simulink model "OpenSeesPy_Simulink"  (R2021a)
settings: Solver=ode8  StartTime=0.0  StopTime=31.2  FixedStep=dtfast  RelTol=1e-3
PreLoadFcn:
  | initializeSimulation;
InitFcn:
  | clear('all');
  | initializeSimulation;
undefined symbols (not defined in the file): adaptive, Area, areaC, asiv, Be, Cl, coef, damperA, damperB, damperC, damperCanon, denfilter, DiscIntNeverNeededParam, dtsim, f, fir_coef, flowCanon, forceCanon, forgfact, frictionA, frictionB, frictionC, gasConstant, Gsnsr_DT, Gsnsr_FT, Kc, ke, kgap, khard, Kp, Kq, kv, learningrate, lengthCanon, massA, massB, massC, massCanon, maxDisplA, maxDisplB, maxDisplC, maxForceC, maxOilVolume, maxVelocA, maxVelocB, maxVelocC, minDisplA, minDisplB, minDisplC, minVelocA, minVelocB, minVelocC, n1siv, n2siv, Ngap, nsiv, numfilter, P_corr_i, precharge, pumpFlow ... (+25)
libraries: simulink x4, instrumentlib x2, dsparch4 x1, sldrtlib x1
(part 1 of 3)
settings Model: Creator=diego.mera  LastModifiedBy=diego.mera
settings SolverCC: PositivePriorityOrder=on
settings OptimizationCC: EnhancedBackFolding=on  PassReuseOutputArgsAs=Individual arguments  ZeroExternalMemoryAtStartup=off  ZeroInternalMemoryAtStartup=off  MaxStackSize=64  OptimizeBlockOrder=speed  DifferentSizesBufferReuse=on  OptimizationCustomize=off  EfficientTunableParamExpr=on
settings DebuggingCC: ParameterTunabilityLossMsg=error
settings HardwareCC: ProdBitPerPointer=32  ProdBitPerSizeT=32  ProdBitPerPtrDiffT=32  ProdLargestAtomicInteger=Long  ProdLargestAtomicFloat=Double  ProdWordSize=32  ProdLongLongMode=on  ProdHWDeviceType=ARM Compatible->ARM Cortex
settings RTWCC: SystemTargetFile=ert.tlc  HardwareBoard=Raspberry Pi  TLCOptions="-aInlineSetEventsForThisBaseRateFcn=TLC_FALSE -aSuppressMultiTaskScheduler=TLC_FALSE  -aRateBasedStepFcn=0"  TemplateMakefile=ert_default_tmf  Toolchain=GNU GCC Embedded Linux  BuildConfiguration=Faster Runs
settings CodeAppCC: ForceParamTrailComments=on  IgnoreCustomStorageClasses=off  OperatorAnnotations=on  SimulinkDataObjDesc=on  SFDataObjDesc=on  InsertBlockDesc=on
settings ERTTargetCC: SupportVariableSizeSignals=on  ExtModeTransport=2  ExtModeStaticAlloc=on  ExtModeMexFile=ext_xcp  ExtModeIntrfLevel=Level2 - Open

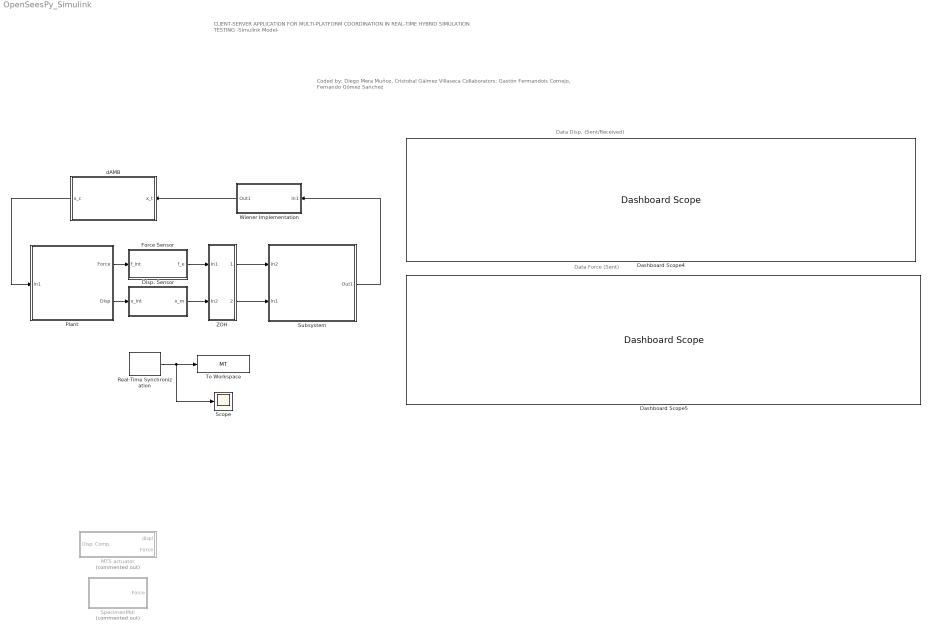
== system OpenSeesPy_Simulink ==
  note: Data Disp. (Sent/Received)
  note: Data Force (Sent)
  note: CLIENT-SERVER APPLICATION FOR MULTI-PLATFORM COORDINATION IN REAL-TIME HYBRID SIMULATION TESTING
      | -Simulink Model-
  note: Coded by: Diego Mera Muñoz, Cristobal Gálmez Villaseca
      | Collaborators: Gastón Fermandois Cornejo, Fernando Gómez Sanchez
  Dashboard Scope4 : DashboardScope  Ymin=-5  Ymax=5
  Dashboard Scope5 : DashboardScope  Ymin=-1.5e-5  Ymax=1e-5
  Disp. Sensor : Subsystem
      mask Display: disp('DISP. SENSOR')
  Force Sensor : Subsystem
      mask Display: disp('FORCE SENSOR')
  MTS actuator : Subsystem  Commented=on
  Plant : Subsystem
      mask Display: disp('PLANT\n(Actuator-ES)')
  Real-Time Synchronization : sldrtlib/Real-Time Synchronization  SampleTime=dtsim  MaxMissedTicks=1000000  ShowMissedTicks=on  YieldWhenWaiting=off
  Scope : Scope
  SpecimenMdl : Subsystem  Commented=on
      mask Display: disp('EXPERIMENTAL\nSUBSTRUCTURE')
  Subsystem : Subsystem
      mask Display: disp('NUMERICAL\nSUBSTRUCTURE')
  To Workspace : ToWorkspace  VariableName=MT  SaveFormat=Timeseries  SampleTime=-1
  Wiener Implementation : Subsystem
      mask Display: disp('MBMRT FILTER')
  ZOH : Subsystem
      mask Display: disp('ZOH')
  dAMB : Subsystem
      mask Display: disp('DISCRETE ADAPTIVE\nMODEL-BASED\nCOMPENSATION')
  wires:
  Subsystem/1(Out1) -> Wiener Implementation/1(In1)
  dAMB/1(x_c) -> Plant/1(In1)
  Real-Time Synchronization/1 -> Scope/1, To Workspace/1
  Wiener Implementation/1(Out1) -> dAMB/1(x_t)
  Plant/1(Force) -> Force Sensor/1(f_int)
  Force Sensor/1("f_e ") -> ZOH/1(In1)
  ZOH/1(Out1) -> Subsystem/1(In2)
  ZOH/2(Out2) -> Subsystem/2(In1)
  Disp. Sensor/1(x_m) -> ZOH/2(In2)
  Plant/2(Disp) -> Disp. Sensor/1(x_int)

== system OpenSeesPy_Simulink/Disp. Sensor ==
  x_int : Inport
  Sensor Noise : simulink/Sources/Band-Limited White Noise  Cov=rms_noise_DT  Ts=dtsim  seed=double(Seed_snr.Seed)
  Sensor Gain LVDT : Gain  Gain=Gsnsr_DT  SaturateOnIntegerOverflow=on  OutDataTypeStr=Inherit: Same as input  ParamDataTypeStr=Inherit: Same as input
  Sum : Sum  Inputs=|++  InputSameDT=on  SaturateOnIntegerOverflow=on  OutDataTypeStr=Inherit: Same as first input
  x_m : Outport
  tag scope: x_m=global
  wires:
  Sensor Noise/1 -> Sum/2
  Sum/1 -> x_m/1, [x_m]  "x_m"
  x_int/1 -> Sensor Gain LVDT/1
  Sensor Gain LVDT/1 -> Sum/1

== system OpenSeesPy_Simulink/Force Sensor ==
  f_int : Inport
  Sensor Noise1 : simulink/Sources/Band-Limited White Noise  Cov=rms_noise_FT  Ts=dtsim  seed=double(Seed_snr.Seed)
  Sensor Gain LOAD CELL : Gain  Gain=Gsnsr_FT  SaturateOnIntegerOverflow=on  OutDataTypeStr=Inherit: Same as input  ParamDataTypeStr=Inherit: Same as input
  Sum1 : Sum  Inputs=|++  InputSameDT=on  SaturateOnIntegerOverflow=on  OutDataTypeStr=Inherit: Same as first input
  "f_e " : Outport
  wires:
  f_int/1 -> Sensor Gain LOAD CELL/1
  Sensor Noise1/1 -> Sum1/2
  Sum1/1 -> "f_e "/1
  Sensor Gain LOAD CELL/1 -> Sum1/1

== system OpenSeesPy_Simulink/MTS actuator ==
  note: Force
  Disp. Comp. : Inport
  Analog Filter Design : dsparch4/Analog Filter Design  method=Butterworth  filttype=Lowpass  N=1  Wlo=20  Whi=80  Rp=2  Rs=40
  Proportional Gain : Gain  Gain=maxForceC/areaC
  Subtract : Sum  Inputs=+-
  accumulators : Subsystem
  dynamic long channel #1 : Subsystem
  dynamic long channel #2 : Subsystem  Commented=on
  dynamic short channel #1 : Subsystem  Commented=on
  dynamic short channel #2 : Subsystem  Commented=on
  static channel #1 : Subsystem  Commented=on
  static channel #2 : Subsystem  Commented=on
  static channel #3 : Subsystem  Commented=on
  static channel #4 : Subsystem  Commented=on
  displ : Outport
  Force : Outport  Port=2
  wires:
  Disp. Comp./1 -> Subtract/1
  Subtract/1 -> Proportional Gain/1
  dynamic long channel #1/3(flow) -> accumulators/1(flow)
  dynamic long channel #1/2(force) -> Analog Filter Design/1
  dynamic long channel #1/1(displ) -> displ/1, Subtract/2
  accumulators/1(press) -> dynamic long channel #1/2(spl press)
  Analog Filter Design/1 -> Force/1
  Proportional Gain/1 -> dynamic long channel #1/1(valve cmd)

== system OpenSeesPy_Simulink/Plant ==
  note: Modeling of Actuator Dynamics
  In1 : Inport
  Actuator : TransferFcn  Denominator=[Vt/(4*Be) Cl]
      mask Display: image(imread('actuator.PNG'));
  Controller : Gain  Gain=Kp
  Gain1 : Gain  Gain=Area
  Gain2 : Gain  Gain=Area
  Scope1 : Scope
  Servovalve Dynamics : TransferFcn  Numerator=[kv]  Denominator=[tauv 1]
      mask Display: image(imread('servo2.PNG'));
  Servovalve Flow : Subsystem
      settings: PortSchema="{\"entries\":[{\"content\":{\"sides\":[{\"content\":{\"connectorIds\":[\"In1\"]},\"type\":\"ConnectorPlacement.EquallySpacedRectSide\",\"uuid\":\"f3a8b7d5-d784-462c-bc82-60644eee5a75\"},{\"content\":{\"connectorIds\":[\"Out1\"],\"side\":\"RIGHT\"},\"type\":\"ConnectorPlacement.EquallySpacedRectSide\",\"uuid\":\"5e6f1f83-a632-4bc9-a761-43cae998e77f\"},{\"content\":{\"connectorIds\":[\"In2\"],\"side\":\"TOP\"},\"type\":\"ConnectorPlacement.EquallySpacedRectSide\",\"uuid\":\"989b0903-e260-4847-946f-0ac5d5e511f7\"}]},\"type\":\"ConnectorPlacement.EquallySpacedConnector\",\"uuid\":\"5619e211-faa3-4076-b1a0-b20862ba0eaa\"}],\"packageUris\":[\"http://schema.mathworks.com/mf0/Connector/19700101\"],\"version\":\"1.0\"}"
      mask Display: image(imread('servo.PNG'));
  Subsystem : Subsystem
      mask Display: disp('EXPERIMENTAL\nSUBSTRUCTURE')
  Sum : Sum  Inputs=|+-
  Sum1 : Sum  Inputs=|+-
  To Workspace : ToWorkspace  VariableName=Force_act  SaveFormat=Timeseries  SampleTime=-1
  Force : Outport
  Disp : Outport  Port=2
  wires:
  Sum/1 -> Controller/1  "e"
  Servovalve Dynamics/1 -> Servovalve Flow/1(xv)  "x_v"
  Gain1/1 -> Sum1/2  "caudal"
  Actuator/1 -> Servovalve Flow/2(pL), Gain2/1  "PL"
  Sum1/1 -> Actuator/1
  Controller/1 -> Servovalve Dynamics/1  "i_c"
  Servovalve Flow/1(QL) -> Sum1/1
  Gain2/1 -> Subsystem/1(F), To Workspace/1, Scope1/1, Force/1  "f_p"
  Subsystem/2(x_m s) -> Gain1/1
  Subsystem/1(x_m) -> Disp/1, Sum/2
  In1/1 -> Sum/1

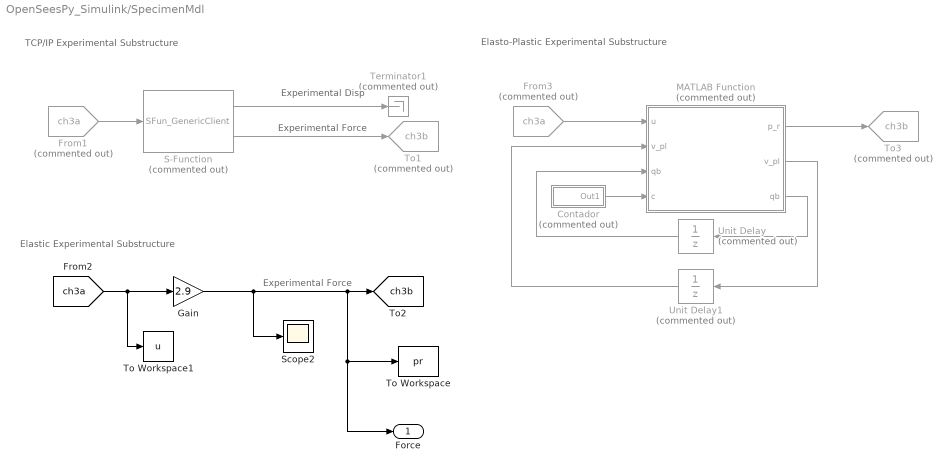
== system OpenSeesPy_Simulink/SpecimenMdl ==
  note: Elasto-Plastic Experimental Substructure
  note: Elastic Experimental Substructure
  note: Experimental Force
  note: Experimental Disp
  note: TCP/IP Experimental Substructure
  note: Experimental Force
  Contador : Subsystem  Commented=on
      mask Display: disp('Contador')
  From1 : From  Commented=on  GotoTag=ch3a  TagVisibility=global
  From3 : From  Commented=on  GotoTag=ch3a  TagVisibility=global
  Gain : Gain  Gain=2.9
  MATLAB Function : MATLAB Function  Commented=on  TreatAsAtomicUnit=on
  S-Function : S-Function  Commented=on  FunctionName=SFun_GenericClient  Parameters=ipAddr,ipPort,dataSize  SFunctionDeploymentMode=off  EnableBusSupport=off  mask(GenericClient Element){ipAddr=127.0.0.1, ipPort=8093, dataSize=256}
      mask prompts: ipAddr "IP Address of Server"; ipPort "IP Port Number of Server"; dataSize "Size of Data Arrays"
      mask Display: disp('GenericClient\nElement');
  Scope2 : Scope
  Terminator1 : Terminator  Commented=on
  To Workspace : ToWorkspace  VariableName=pr  SaveFormat=Timeseries  SampleTime=-1
  To Workspace1 : ToWorkspace  VariableName=u  SaveFormat=Timeseries  SampleTime=-1
  To1 : Goto  Commented=on  GotoTag=ch3b  TagVisibility=global
  To3 : Goto  Commented=on  GotoTag=ch3b  TagVisibility=global
  Unit Delay : UnitDelay  Commented=on  SampleTime=-1  HasFrameUpgradeWarning=on
  Unit Delay1 : UnitDelay  Commented=on  SampleTime=-1  HasFrameUpgradeWarning=on
  Force : Outport
  tag scope: ch3b=global
  wires:
  [ch3a] -> To Workspace1/1, Gain/1
  Gain/1 -> To Workspace/1, Force/1, [ch3b], Scope2/1
  From3/1 -> MATLAB Function/1(u)
  MATLAB Function/3(qb) -> Unit Delay/1
  MATLAB Function/1(p_r) -> To3/1
  Unit Delay/1 -> MATLAB Function/3("qb ")
  Contador/1(Out1) -> MATLAB Function/4(c)
  MATLAB Function/2(v_pl) -> Unit Delay1/1
  Unit Delay1/1 -> MATLAB Function/2("v_pl ")
  From1/1 -> S-Function/1
  S-Function/2 -> To1/1
  S-Function/1 -> Terminator1/1

== system OpenSeesPy_Simulink/Subsystem ==
  In2 : Inport
  In1 : Inport  Port=2
  TCP/IP Receive5 : instrumentlib/TCP//IP Receive  Priority=1  Host=127.0.0.1  Port=8090  DataSize=1  EnableBlockingMode=off  Timeout=10  SampleTime=dtsim  DataType=double  ByteOrder=BigEndian  ASCIIFormatting=%f,  Terminator=LF
  TCP/IP Send5 : instrumentlib/TCP//IP Send  Priority=2  Host=127.0.0.1  Port=8090  EnableBlockingMode=off  Timeout=0.02  ByteOrder=BigEndian  TransferDelay=on
  Terminator : Terminator
  To Workspace : ToWorkspace  VariableName=Disp_Num  SaveFormat=Timeseries  SampleTime=-1
  Out1 : Outport
  wires:
  In1/1 -> Terminator/1
  In2/1 -> TCP/IP Send5/1
  TCP/IP Receive5/1 -> To Workspace/1, Out1/1

== system OpenSeesPy_Simulink/Wiener Implementation ==
  In1 : Inport
  Prediction_Adaptive_Fixed : Subsystem
      mask Display: disp('PREDICTION\n(Adaptive/Fixed w)')
  Test3 : Subsystem
      mask Display: disp('MONOMIAL\nINTERPOLATION')
  To Workspace : ToWorkspace  VariableName=adaptive_parameters  SaveFormat=Timeseries  SampleTime=-1
  Out1 : Outport
  wires:
  Test3/1(Out1) -> Out1/1
  In1/1 -> Prediction_Adaptive_Fixed/1(In1)
  Prediction_Adaptive_Fixed/2(Out2) -> To Workspace/1
  Prediction_Adaptive_Fixed/1(Out1) -> Test3/1(In1)

== system OpenSeesPy_Simulink/ZOH ==
  In1 : Inport
  In2 : Inport  Port=2
  Rate Transition : RateTransition  OutPortSampleTime=dtsim
  Rate Transition1 : RateTransition  OutPortSampleTime=dtsim
  Out1 : Outport
  Out2 : Outport  Port=2
  wires:
  In1/1 -> Rate Transition/1  "Force_Num"
  In2/1 -> Rate Transition1/1  "Disp_Num"
  Rate Transition/1 -> Out1/1
  Rate Transition1/1 -> Out2/1

== system OpenSeesPy_Simulink/dAMB ==
  x_t : Inport
  Discrete Transfer Fcn : DiscreteTransferFcn  Numerator=[numfilter]  Denominator=[denfilter]
  Discrete Transfer Fcn1 : DiscreteTransferFcn  Numerator=[numfilter]  Denominator=[denfilter]
  Dot Product : DotProduct  InputSameDT=on  OutDataTypeStr=Inherit: Inherit via internal rule
  Gain : Gain  Gain=0.0254
  Gain1 : Gain  Gain=0.0254
  Gain2 : Gain  Gain=39.3701
  RLS : Subsystem
  Tapped Delay : simulink/Discrete/Tapped Delay  vinit=0.0  samptime=-1  NumDelays=fir_coef-1  DelayOrder=Newest  includeCurrent=on
  Tapped Delay1 : simulink/Discrete/Tapped Delay  vinit=0.0  samptime=-1  NumDelays=fir_coef-1  DelayOrder=Newest  includeCurrent=on
  To Workspace : ToWorkspace  VariableName=x_t  SaveFormat=Timeseries  SampleTime=-1
  Unit Delay1 : UnitDelay  SampleTime=-1  HasFrameUpgradeWarning=on
  Unit Delay3 : UnitDelay  SampleTime=-1  HasFrameUpgradeWarning=on
  x_c : Outport  VectorParamsAs1DForOutWhenUnconnected=off
  wires:
  Gain1/1 -> Unit Delay3/1
  Gain/1 -> Tapped Delay/1
  Tapped Delay/1 -> Dot Product/1
  x_t/1 -> To Workspace/1, Gain/1
  Discrete Transfer Fcn/1 -> Tapped Delay1/1
  Discrete Transfer Fcn1/1 -> RLS/2(u)
  Tapped Delay1/1 -> RLS/1(xm)
  RLS/1(dAMB) -> Dot Product/2
  Unit Delay3/1 -> Discrete Transfer Fcn/1
  Unit Delay1/1 -> Discrete Transfer Fcn1/1
  Dot Product/1 -> Gain2/1, Unit Delay1/1
  Gain2/1 -> x_c/1
  [x_m] -> Gain1/1

== system OpenSeesPy_Simulink/MTS actuator/accumulators ==
  flow : Inport
  Sum : Sum  Inputs=+-|  InputSameDT=on  SaturateOnIntegerOverflow=on  OutDataTypeStr=Inherit: Same as first input
  Sum1 : Sum  Inputs=+-|  InputSameDT=on  SaturateOnIntegerOverflow=on  OutDataTypeStr=Inherit: Same as first input
  bottle volume : Constant  Value=volume*volumeCanon
  flowCanon : Gain  Gain=flowCanon  SaturateOnIntegerOverflow=on  OutDataTypeStr=Inherit: Same as input  ParamDataTypeStr=Inherit: Same as input
  gas constant : Constant  Value=gasConstant
  initial condition : UnitDelay  InitialCondition=supplyPress  SampleTime=-1  HasFrameUpgradeWarning=on
  integrator : DiscreteIntegrator  InitialCondition=maxOilVolume*volumeCanon  SampleTime=1/4000  LimitOutput=on  UpperSaturationLimit=maxOilVolume*volumeCanon  LowerSaturationLimit=0  ICPrevOutput=DiscIntNeverNeededParam  ICPrevScaledInput=DiscIntNeverNeededParam
  power : Math  Operator=pow  SignedPower=on  SaturateOnIntegerOverflow=on
  precharge : Gain  Gain=precharge  SaturateOnIntegerOverflow=on  OutDataTypeStr=Inherit: Same as input  ParamDataTypeStr=Inherit: Same as input
  pump flow : Constant  Value=pumpFlow
  quotient : Product  Inputs=*/  InputSameDT=on  SaturateOnIntegerOverflow=on  OutDataTypeStr=Inherit: Same as first input
  press : Outport
  wires:
  initial condition/1 -> press/1
  flowCanon/1 -> integrator/1
  flow/1 -> Sum/2
  integrator/1 -> Sum1/2  "current oil volume"
  quotient/1 -> power/1
  Sum1/1 -> quotient/2  "current gas volume"
  precharge/1 -> initial condition/1
  power/1 -> precharge/1
  gas constant/1 -> power/2
  bottle volume/1 -> quotient/1, Sum1/1
  Sum/1 -> flowCanon/1
  pump flow/1 -> Sum/1

== system OpenSeesPy_Simulink/MTS actuator/dynamic long channel #1 ==
  valve cmd : Inport
  spl press : Inport  Port=2
  actuator/valve model : Subsystem  mask(Inverse Actuator){}
  payload : Subsystem
  return pressure : Constant  Value=returnPress
  displ : Outport
  force : Outport  Port=2
  flow : Outport  Port=3
  wires:
  actuator/valve model/1(force) -> payload/1(force), force/1
  actuator/valve model/2(flow) -> flow/1
  spl press/1 -> actuator/valve model/4(spl press)
  return pressure/1 -> actuator/valve model/5(rtn press)
  valve cmd/1 -> actuator/valve model/1(cmd)
  payload/1(displ) -> actuator/valve model/2(displ), displ/1
  payload/2(veloc) -> actuator/valve model/3(veloc)

== system OpenSeesPy_Simulink/MTS actuator/dynamic long channel #2 ==
  valve cmd : Inport
  spl press : Inport  Port=2
  actuator/valve model : Subsystem  mask(Inverse Actuator){}
  payload : Subsystem
  return pressure : Constant  Value=returnPress
  displ : Outport
  force : Outport  Port=2
  dpforce : Outport  Port=3
  flow : Outport  Port=4
  wires:
  payload/2(veloc) -> actuator/valve model/3(veloc)
  payload/1(displ) -> displ/1, actuator/valve model/2(displ)
  valve cmd/1 -> actuator/valve model/1(cmd)
  return pressure/1 -> actuator/valve model/5(rtn press)
  spl press/1 -> actuator/valve model/4(spl press)
  actuator/valve model/2(flow) -> flow/1
  actuator/valve model/1(force) -> payload/1(force), force/1, dpforce/1

== system OpenSeesPy_Simulink/MTS actuator/dynamic short channel #1 ==
  valve cmd : Inport
  spl press : Inport  Port=2
  actuator/valve model : Subsystem  mask(Inverse Actuator){}
  payload : Subsystem
  return pressure : Constant  Value=returnPress
  displ : Outport
  force : Outport  Port=2
  dpforce : Outport  Port=3
  flow : Outport  Port=4
  wires:
  payload/2(veloc) -> actuator/valve model/3(veloc)
  payload/1(displ) -> displ/1, actuator/valve model/2(displ)
  valve cmd/1 -> actuator/valve model/1(cmd)
  return pressure/1 -> actuator/valve model/5(rtn press)
  spl press/1 -> actuator/valve model/4(spl press)
  actuator/valve model/2(flow) -> flow/1
  actuator/valve model/1(force) -> payload/1(force), force/1, dpforce/1

== system OpenSeesPy_Simulink/MTS actuator/dynamic short channel #2 ==
  valve cmd : Inport
  spl press : Inport  Port=2
  actuator/valve model : Subsystem  mask(Inverse Actuator){}
  payload : Subsystem
  return pressure : Constant  Value=returnPress
  displ : Outport
  force : Outport  Port=2
  dpforce : Outport  Port=3
  flow : Outport  Port=4
  wires:
  payload/2(veloc) -> actuator/valve model/3(veloc)
  payload/1(displ) -> displ/1, actuator/valve model/2(displ)
  valve cmd/1 -> actuator/valve model/1(cmd)
  return pressure/1 -> actuator/valve model/5(rtn press)
  spl press/1 -> actuator/valve model/4(spl press)
  actuator/valve model/2(flow) -> flow/1
  actuator/valve model/1(force) -> payload/1(force), force/1, dpforce/1

== system OpenSeesPy_Simulink/MTS actuator/static channel #1 ==
  valve cmd : Inport
  spl press : Inport  Port=2
  actuator/valve model : Subsystem  mask(Inverse Actuator){}
  payload : Subsystem
  return pressure : Constant  Value=returnPress
  displ : Outport
  force : Outport  Port=2
  dpforce : Outport  Port=3
  flow : Outport  Port=4
  wires:
  actuator/valve model/1(force) -> payload/1(force), dpforce/1, force/1
  actuator/valve model/2(flow) -> flow/1
  spl press/1 -> actuator/valve model/4(spl press)
  return pressure/1 -> actuator/valve model/5(rtn press)
  valve cmd/1 -> actuator/valve model/1(cmd)
  payload/1(displ) -> actuator/valve model/2(displ), displ/1
  payload/2(veloc) -> actuator/valve model/3(veloc)

== system OpenSeesPy_Simulink/MTS actuator/static channel #2 ==
  valve cmd : Inport
  spl press : Inport  Port=2
  actuator/valve model : Subsystem  mask(Inverse Actuator){}
  payload : Subsystem
  return pressure : Constant  Value=returnPress
  displ : Outport
  force : Outport  Port=2
  dpforce : Outport  Port=3
  flow : Outport  Port=4
  wires:
  payload/2(veloc) -> actuator/valve model/3(veloc)
  payload/1(displ) -> displ/1, actuator/valve model/2(displ)
  valve cmd/1 -> actuator/valve model/1(cmd)
  return pressure/1 -> actuator/valve model/5(rtn press)
  spl press/1 -> actuator/valve model/4(spl press)
  actuator/valve model/2(flow) -> flow/1
  actuator/valve model/1(force) -> payload/1(force), force/1, dpforce/1

== system OpenSeesPy_Simulink/MTS actuator/static channel #3 ==
  valve cmd : Inport
  spl press : Inport  Port=2
  actuator/valve model : Subsystem  mask(Inverse Actuator){}
  payload : Subsystem
  return pressure : Constant  Value=returnPress
  displ : Outport
  force : Outport  Port=2
  dpforce : Outport  Port=3
  flow : Outport  Port=4
  wires:
  actuator/valve model/1(force) -> payload/1(force), dpforce/1, force/1
  actuator/valve model/2(flow) -> flow/1
  spl press/1 -> actuator/valve model/4(spl press)
  return pressure/1 -> actuator/valve model/5(rtn press)
  valve cmd/1 -> actuator/valve model/1(cmd)
  payload/1(displ) -> actuator/valve model/2(displ), displ/1
  payload/2(veloc) -> actuator/valve model/3(veloc)

== system OpenSeesPy_Simulink/MTS actuator/static channel #4 ==
  valve cmd : Inport
  spl press : Inport  Port=2
  actuator/valve model : Subsystem  mask(Inverse Actuator){}
  payload : Subsystem
  return pressure : Constant  Value=returnPress
  displ : Outport
  force : Outport  Port=2
  dpforce : Outport  Port=3
  flow : Outport  Port=4
  wires:
  payload/2(veloc) -> actuator/valve model/3(veloc)
  payload/1(displ) -> displ/1, actuator/valve model/2(displ)
  valve cmd/1 -> actuator/valve model/1(cmd)
  return pressure/1 -> actuator/valve model/5(rtn press)
  spl press/1 -> actuator/valve model/4(spl press)
  actuator/valve model/2(flow) -> flow/1
  actuator/valve model/1(force) -> payload/1(force), force/1, dpforce/1

== system OpenSeesPy_Simulink/Plant/Servovalve Flow ==
  xv : Inport
  pL : Inport  Port=2
  Gain : Gain  Gain=Kq
  Gain1 : Gain  Gain=Kc
  Subtract : Sum  Inputs=+-
  QL : Outport
  wires:
  Gain1/1 -> Subtract/2
  pL/1 -> Gain1/1
  Subtract/1 -> QL/1
  Gain/1 -> Subtract/1
  xv/1 -> Gain/1

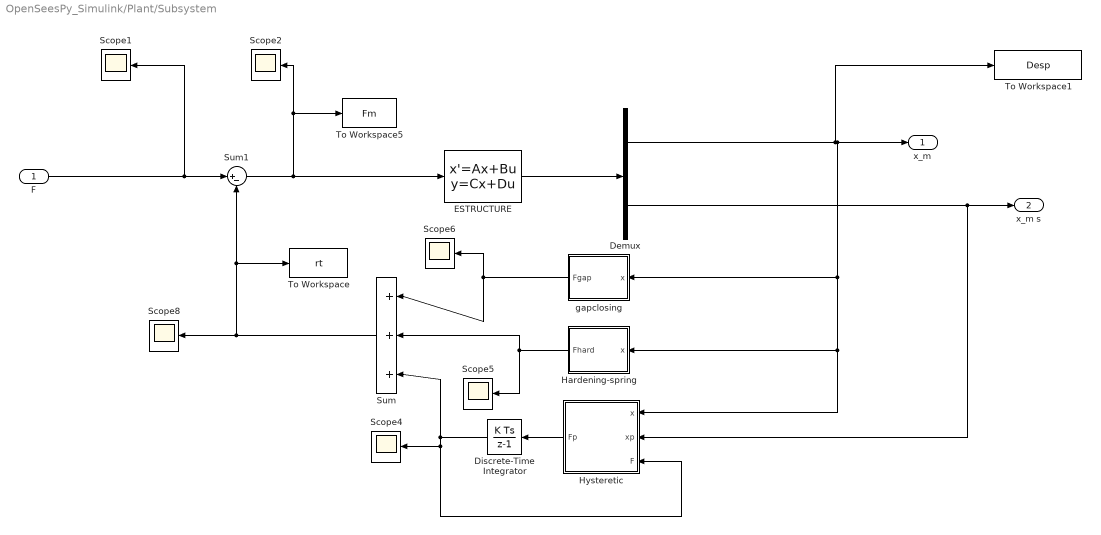
== system OpenSeesPy_Simulink/Plant/Subsystem ==
  F : Inport
  Demux : Demux  Outputs=2
  Discrete-Time Integrator : DiscreteIntegrator  SampleTime=-1  ICPrevOutput=DiscIntNeverNeededParam  ICPrevScaledInput=DiscIntNeverNeededParam
  ESTRUCTURE : StateSpace  A=ssAe  B=ssBe  C=ssCe  D=ssDe  InitialCondition=0
  Hardening-spring : Subsystem
  Hysteretic : Subsystem
  Scope{1..2,4..6,8} (6 alike) : Scope
  Sum : Sum  Inputs=|+++
  Sum1 : Sum  Inputs=|+-
  To Workspace : ToWorkspace  VariableName=rt  SaveFormat=Timeseries  SampleTime=-1
  To Workspace1 : ToWorkspace  VariableName=Desp  SaveFormat=Timeseries  SampleTime=-1
  To Workspace5 : ToWorkspace  VariableName=Fm  SaveFormat=Timeseries  SampleTime=-1
  gapclosing : Subsystem
  x_m : Outport  VectorParamsAs1DForOutWhenUnconnected=off
  x_m s : Outport  Port=2  VectorParamsAs1DForOutWhenUnconnected=off
  wires:
  Sum/1 -> To Workspace/1, Sum1/2, Scope8/1
  gapclosing/1(Fgap) -> Scope6/1, Sum/1
  Sum1/1 -> Scope2/1, To Workspace5/1, ESTRUCTURE/1
  Discrete-Time Integrator/1 -> Sum/3, Scope4/1, Hysteretic/3(F)
  Hardening-spring/1(Fhard) -> Scope5/1, Sum/2
  Demux/1 -> To Workspace1/1, x_m/1, Hardening-spring/1(x), Hysteretic/1(x), gapclosing/1(x)
  Hysteretic/1(Fp) -> Discrete-Time Integrator/1
  Demux/2 -> x_m s/1, Hysteretic/2(xp)
  ESTRUCTURE/1 -> Demux/1
  F/1 -> Scope1/1, Sum1/1

== system OpenSeesPy_Simulink/SpecimenMdl/Contador ==
  Add : Sum
  Constant1 : Constant
  Unit Delay : UnitDelay  SampleTime=-1  HasFrameUpgradeWarning=on
  Out1 : Outport
  wires:
  Unit Delay/1 -> Add/2
  Constant1/1 -> Add/1
  Add/1 -> Out1/1, Unit Delay/1

== system OpenSeesPy_Simulink/Wiener Implementation/Prediction_Adaptive_Fixed ==
  In1 : Inport
  Constant : Constant  Value=learningrate*adaptive
  Contador : Subsystem
      mask Display: disp('Contador')
  Discrete FIR Filter : DiscreteFir  CoefSource=Input port  SampleTime=dtsim
      settings: InputPortMap=u0,u1
  If : If  IfExpression=u1 <2
  If Action Subsystem : Subsystem  TreatAsAtomicUnit=on
  If Action Subsystem1 : Subsystem  TreatAsAtomicUnit=on
  Merge : Merge
  Unit Delay1 : UnitDelay  SampleTime=-1  HasFrameUpgradeWarning=on
  Out1 : Outport
  Out2 : Outport  Port=2
  wires:
  If Action Subsystem/1(W_new) -> Merge/1
  In1/1 -> Discrete FIR Filter/1, If Action Subsystem/1(Disp), If Action Subsystem1/1(Disp)
  If Action Subsystem1/1(W_new) -> Merge/2
  If/1 -> If Action Subsystem/Action
  Unit Delay1/1 -> If Action Subsystem1/2(W_prev)
  If/2 -> If Action Subsystem1/Action
  Contador/1(Out1) -> If/1
  Constant/1 -> If Action Subsystem1/3(lambda), If Action Subsystem/2(lambda)
  Discrete FIR Filter/1 -> [A], Out1/1
  [A] -> If Action Subsystem/3(Disp_Pred)
  [A] -> If Action Subsystem1/4(Disp_Pred)
  Merge/1 -> Discrete FIR Filter/2, Out2/1, Unit Delay1/1

== system OpenSeesPy_Simulink/Wiener Implementation/Test3 ==
  In1 : Inport
  Buffer : Buffer  N=4  V=3  OutputFrames=off
  Constant6 : Constant  Value=V1
  Product1 : Product  Multiplication=Matrix(*)
  Product2 : Product  Multiplication=Matrix(*)
  Subsystem : Subsystem
  Unbuffer2 : Unbuffer
  Out1 : Outport
  wires:
  Product2/1 -> Product1/2
  Constant6/1 -> Product2/1
  Unbuffer2/1 -> Out1/1
  In1/1 -> Buffer/1
  Product1/1 -> Unbuffer2/1
  Subsystem/1(a) -> Product1/1
  Buffer/1 -> Product2/2

== system OpenSeesPy_Simulink/dAMB/RLS ==
  xm : Inport
  u : Inport  Port=2
  Constant6 : Constant  Value=forgfact
  Delay1 : Delay  DelayLength=1  InitialCondition=P_corr_i
  Delay2 : Delay  DelayLength=1  InitialCondition=dAMB_i'
  RLS : MATLAB Function  TreatAsAtomicUnit=on
  To Workspace : ToWorkspace  VariableName=dAMB  SaveFormat=Timeseries  SampleTime=-1
  To Workspace1 : ToWorkspace  VariableName=P_corr  SaveFormat=Timeseries  SampleTime=-1
  dAMB : Outport  VectorParamsAs1DForOutWhenUnconnected=off
  wires:
  xm/1 -> RLS/1(xm)
  Delay2/1 -> RLS/4(dAMB_a)
  u/1 -> RLS/2(u)
  RLS/2(P_corr) -> To Workspace1/1, Delay1/1
  Delay1/1 -> RLS/5(P_corr_a)
  Constant6/1 -> RLS/3(forgfact)
  RLS/1(dAMB) -> Delay2/1, dAMB/1, To Workspace/1

== system OpenSeesPy_Simulink/MTS actuator/dynamic long channel #1/actuator//valve model ==
  note: Parameter vector:
      | 1:   oil bulk modulus (force/displ^2)
      | 2:   servovalve delay (sec)
      | 3:   servovalve overlap
      | 4:   rated pressure (force/displ^2)
      | 5:   rated flow at rated pressure (displ^3/sec)
      | 6:   nominal flow at rated pressure (displ^3/sec)
      | 7:   actuator piston area 1 (displ^2)
      | 8:   actuator piston area 2 (displ^2)
      | 9:   actuator usable stroke 1 (displ)
      | 10: actuator usable stroke 2 (displ)
      | 11: actuator end cushion length 1 (displ)
      | 12: actuator end cushion length 2 (displ)
      | 13: actuator parasitic damping factor
      | 14: cross-chamber leakage factor (flow/press)
      | 15: ratio port openings according to area
      | 16: sample period (sec)
      |
      | Conversion factors used for converting
      | signals from external (user) to internal
      | (canonical) units:
      |
      | 17: displacement
      | 18: velocity
      | 19: force
      | 20: pressure
      | 21: flow
  note: Auxiliary diagnostic output vector:
      | 1:   valve opening
      | 2:   C1 pressure
      | 3:   C2 pressure
      | 4:   delta pressure
      | 5:   force
      | 6:   velocity
      | 7:   C1 flow
      | 8:   C2 flow
      | 9:   total flow
      | 10: kinematic flow
      | 11: compressibility flow
      | 12: leakage flow
  note: Note: "1" and "2" denote actuator
      | cylinders on either side of the
      | actuator piston.  With positive
      | valve drive, oil is ported into
      | cylinder 1, resulting in positive
      | displacement.
  cmd : Inport
  displ : Inport  Port=2
  veloc : Inport  Port=3
  spl press : Inport  Port=4
  rtn press : Inport  Port=5
  abs : Abs  SaturateOnIntegerOverflow=on
  actuator : S-Function  FunctionName=actuator  Parameters=actParamsB  SFunctionDeploymentMode=off  EnableBusSupport=off
  total flow sel : Selector  InputPortWidth=12  IndexOptions=Index vector (dialog)  Indices=9  OutputSizes=1
  force : Outport
  flow : Outport  Port=2
  wires:
  abs/1 -> flow/1
  actuator/2 -> total flow sel/1
  total flow sel/1 -> abs/1
  spl press/1 -> actuator/4
  rtn press/1 -> actuator/5
  cmd/1 -> actuator/1
  actuator/1 -> force/1
  displ/1 -> actuator/2
  veloc/1 -> actuator/3

== system OpenSeesPy_Simulink/MTS actuator/dynamic long channel #1/payload ==
  force : Inport
  Sum : Sum  Inputs=+----  InputSameDT=on  SaturateOnIntegerOverflow=on  OutDataTypeStr=Inherit: Same as first input
  damper : Gain  Gain=damperB*damperCanon  SaturateOnIntegerOverflow=on  OutDataTypeStr=Inherit: Same as input  ParamDataTypeStr=Inherit: Same as input
  div : Product  Inputs=*/  InputSameDT=on  SaturateOnIntegerOverflow=on  OutDataTypeStr=Inherit: Same as first input
  double integrator : Subsystem
  friction : Subsystem  mask{friction=frictionB*forceCanon, yieldDispl=yieldDisplB*lengthCanon, hysteresis=0}
      mask prompts: friction "Sliding friction"; yieldDispl "Equiv. yield displacement (in)"; hysteresis "Hysteresis constant"
  mass : Constant  Value=massB*massCanon
  static force : Constant  Value=staticForceB*forceCanon
  term1 : Terminator
  unit dly : UnitDelay  SampleTime=-1  HasFrameUpgradeWarning=on
  unit dly1 : UnitDelay  SampleTime=-1  HasFrameUpgradeWarning=on
  veloc units : Gain  Gain=1/velocCanon  SaturateOnIntegerOverflow=on  OutDataTypeStr=Inherit: Same as input  ParamDataTypeStr=Inherit: Same as input
  displ : Outport
  veloc : Outport  Port=2
  tag scope: ch3a=global
  wires:
  unit dly1/1 -> damper/1
  unit dly/1 -> [ch3a]
  [ch3b] -> Sum/3  "spring force"
  damper/1 -> Sum/4  "damper force"
  static force/1 -> Sum/5  "static force"
  double integrator/2(veloc) -> unit dly1/1, friction/1(veloc), veloc units/1
  double integrator/1(displ) -> unit dly/1, displ/1
  div/1 -> double integrator/1(accel)
  double integrator/3(acc) -> term1/1
  mass/1 -> div/2
  force/1 -> Sum/1  "total force"
  Sum/1 -> div/1  "inertial force"
  veloc units/1 -> veloc/1
  friction/1(force) -> Sum/2  "friction force"

== system OpenSeesPy_Simulink/MTS actuator/dynamic long channel #2/actuator//valve model ==
  note: Parameter vector:
      | 1:   oil bulk modulus (force/displ^2)
      | 2:   servovalve delay (sec)
      | 3:   servovalve overlap
      | 4:   rated pressure (force/displ^2)
      | 5:   rated flow at rated pressure (displ^3/sec)
      | 6:   nominal flow at rated pressure (displ^3/sec)
      | 7:   actuator piston area 1 (displ^2)
      | 8:   actuator piston area 2 (displ^2)
      | 9:   actuator usable stroke 1 (displ)
      | 10: actuator usable stroke 2 (displ)
      | 11: actuator end cushion length 1 (displ)
      | 12: actuator end cushion length 2 (displ)
      | 13: actuator parasitic damping factor
      | 14: cross-chamber leakage factor (flow/press)
      | 15: ratio port openings according to area
      | 16: sample period (sec)
      |
      | Conversion factors used for converting
      | signals from external (user) to internal
      | (canonical) units:
      |
      | 17: displacement
      | 18: velocity
      | 19: force
      | 20: pressure
      | 21: flow
  note: Note: "1" and "2" denote actuator
      | cylinders on either side of the
      | actuator piston.  With positive
      | valve drive, oil is ported into
      | cylinder 1, resulting in positive
      | displacement.
  note: Auxiliary diagnostic output vector:
      | 1:   valve opening
      | 2:   C1 pressure
      | 3:   C2 pressure
      | 4:   delta pressure
      | 5:   force
      | 6:   velocity
      | 7:   C1 flow
      | 8:   C2 flow
      | 9:   total flow
      | 10: kinematic flow
      | 11: compressibility flow
      | 12: leakage flow
  cmd : Inport
  displ : Inport  Port=2
  veloc : Inport  Port=3
  spl press : Inport  Port=4
  rtn press : Inport  Port=5
  abs : Abs  SaturateOnIntegerOverflow=on
  actuator : S-Function  FunctionName=actuator  Parameters=actParamsB  SFunctionDeploymentMode=off  EnableBusSupport=off
  total flow sel : Selector  InputPortWidth=12  IndexOptions=Index vector (dialog)  Indices=9  OutputSizes=1
  force : Outport
  flow : Outport  Port=2
  wires:
  veloc/1 -> actuator/3
  displ/1 -> actuator/2
  actuator/1 -> force/1
  cmd/1 -> actuator/1
  rtn press/1 -> actuator/5
  spl press/1 -> actuator/4
  total flow sel/1 -> abs/1
  actuator/2 -> total flow sel/1
  abs/1 -> flow/1

== system OpenSeesPy_Simulink/MTS actuator/dynamic long channel #2/payload ==
  force : Inport
  Sum : Sum  Inputs=+----  InputSameDT=on  SaturateOnIntegerOverflow=on  OutDataTypeStr=Inherit: Same as first input
  damper : Gain  Gain=damperB*damperCanon  SaturateOnIntegerOverflow=on  OutDataTypeStr=Inherit: Same as input  ParamDataTypeStr=Inherit: Same as input
  div : Product  Inputs=*/  InputSameDT=on  SaturateOnIntegerOverflow=on  OutDataTypeStr=Inherit: Same as first input
  double integrator : Subsystem
  friction : Subsystem  mask{friction=frictionB*forceCanon, yieldDispl=yieldDisplB*lengthCanon, hysteresis=0}
      mask prompts: friction "Sliding friction"; yieldDispl "Equiv. yield displacement (in)"; hysteresis "Hysteresis constant"
  mass : Constant  Value=massB*massCanon
  static force : Constant  Value=staticForceB*forceCanon
  term1 : Terminator
  unit dly : UnitDelay  SampleTime=-1  HasFrameUpgradeWarning=on
  unit dly1 : UnitDelay  SampleTime=-1  HasFrameUpgradeWarning=on
  veloc units : Gain  Gain=1/velocCanon  SaturateOnIntegerOverflow=on  OutDataTypeStr=Inherit: Same as input  ParamDataTypeStr=Inherit: Same as input
  displ : Outport
  veloc : Outport  Port=2
  tag scope: ch4a=global
  wires:
  unit dly/1 -> [ch4a]
  [ch4b] -> Sum/3  "spring force"
  unit dly1/1 -> damper/1
  damper/1 -> Sum/4  "damper force"
  static force/1 -> Sum/5  "static force"
  double integrator/2(veloc) -> unit dly1/1, friction/1(veloc), veloc units/1
  double integrator/1(displ) -> unit dly/1, displ/1
  div/1 -> double integrator/1(accel)
  double integrator/3(acc) -> term1/1
  mass/1 -> div/2
  force/1 -> Sum/1  "total force"
  Sum/1 -> div/1  "inertial force"
  veloc units/1 -> veloc/1
  friction/1(force) -> Sum/2  "friction force"

== system OpenSeesPy_Simulink/MTS actuator/dynamic short channel #1/actuator//valve model ==
  note: Parameter vector:
      | 1:   oil bulk modulus (force/displ^2)
      | 2:   servovalve delay (sec)
      | 3:   servovalve overlap
      | 4:   rated pressure (force/displ^2)
      | 5:   rated flow at rated pressure (displ^3/sec)
      | 6:   nominal flow at rated pressure (displ^3/sec)
      | 7:   actuator piston area 1 (displ^2)
      | 8:   actuator piston area 2 (displ^2)
      | 9:   actuator usable stroke 1 (displ)
      | 10: actuator usable stroke 2 (displ)
      | 11: actuator end cushion length 1 (displ)
      | 12: actuator end cushion length 2 (displ)
      | 13: actuator parasitic damping factor
      | 14: cross-chamber leakage factor (flow/press)
      | 15: ratio port openings according to area
      | 16: sample period (sec)
      |
      | Conversion factors used for converting
      | signals from external (user) to internal
      | (canonical) units:
      |
      | 17: displacement
      | 18: velocity
      | 19: force
      | 20: pressure
      | 21: flow
  note: Note: "1" and "2" denote actuator
      | cylinders on either side of the
      | actuator piston.  With positive
      | valve drive, oil is ported into
      | cylinder 1, resulting in positive
      | displacement.
  note: Auxiliary diagnostic output vector:
      | 1:   valve opening
      | 2:   C1 pressure
      | 3:   C2 pressure
      | 4:   delta pressure
      | 5:   force
      | 6:   velocity
      | 7:   C1 flow
      | 8:   C2 flow
      | 9:   total flow
      | 10: kinematic flow
      | 11: compressibility flow
      | 12: leakage flow
  cmd : Inport
  displ : Inport  Port=2
  veloc : Inport  Port=3
  spl press : Inport  Port=4
  rtn press : Inport  Port=5
  abs : Abs  SaturateOnIntegerOverflow=on
  actuator : S-Function  FunctionName=actuator  Parameters=actParamsA  SFunctionDeploymentMode=off  EnableBusSupport=off
  total flow sel : Selector  InputPortWidth=12  IndexOptions=Index vector (dialog)  Indices=9  OutputSizes=1
  force : Outport
  flow : Outport  Port=2
  wires:
  veloc/1 -> actuator/3
  displ/1 -> actuator/2
  actuator/1 -> force/1
  cmd/1 -> actuator/1
  rtn press/1 -> actuator/5
  spl press/1 -> actuator/4
  total flow sel/1 -> abs/1
  actuator/2 -> total flow sel/1
  abs/1 -> flow/1

== system OpenSeesPy_Simulink/MTS actuator/dynamic short channel #1/payload ==
  force : Inport
  Sum : Sum  Inputs=+----  InputSameDT=on  SaturateOnIntegerOverflow=on  OutDataTypeStr=Inherit: Same as first input
  damper : Gain  Gain=damperA*damperCanon  SaturateOnIntegerOverflow=on  OutDataTypeStr=Inherit: Same as input  ParamDataTypeStr=Inherit: Same as input
  div : Product  Inputs=*/  InputSameDT=on  SaturateOnIntegerOverflow=on  OutDataTypeStr=Inherit: Same as first input
  double integrator : Subsystem
  friction : Subsystem  mask{friction=frictionA*forceCanon, yieldDispl=yieldDisplA*lengthCanon, hysteresis=0}
      mask prompts: friction "Sliding friction"; yieldDispl "Equiv. yield displacement (in)"; hysteresis "Hysteresis constant"
  mass : Constant  Value=massA*massCanon
  static force : Constant  Value=staticForceA*forceCanon
  term1 : Terminator
  unit dly : UnitDelay  SampleTime=-1  HasFrameUpgradeWarning=on
  unit dly1 : UnitDelay  SampleTime=-1  HasFrameUpgradeWarning=on
  veloc units : Gain  Gain=1/velocCanon  SaturateOnIntegerOverflow=on  OutDataTypeStr=Inherit: Same as input  ParamDataTypeStr=Inherit: Same as input
  displ : Outport
  veloc : Outport  Port=2
  tag scope: ch1a=global
  wires:
  unit dly1/1 -> damper/1
  unit dly/1 -> [ch1a]
  double integrator/1(displ) -> displ/1, unit dly/1
  [ch1b] -> Sum/3  "spring force"
  double integrator/2(veloc) -> friction/1(veloc), unit dly1/1, veloc units/1
  damper/1 -> Sum/4  "damper force"
  static force/1 -> Sum/5  "static force"
  div/1 -> double integrator/1(accel)
  double integrator/3(acc) -> term1/1
  mass/1 -> div/2
  force/1 -> Sum/1  "total force"
  Sum/1 -> div/1  "inertial force"
  veloc units/1 -> veloc/1
  friction/1(force) -> Sum/2  "friction force"

== system OpenSeesPy_Simulink/MTS actuator/dynamic short channel #2/actuator//valve model ==
  note: Parameter vector:
      | 1:   oil bulk modulus (force/displ^2)
      | 2:   servovalve delay (sec)
      | 3:   servovalve overlap
      | 4:   rated pressure (force/displ^2)
      | 5:   rated flow at rated pressure (displ^3/sec)
      | 6:   nominal flow at rated pressure (displ^3/sec)
      | 7:   actuator piston area 1 (displ^2)
      | 8:   actuator piston area 2 (displ^2)
      | 9:   actuator usable stroke 1 (displ)
      | 10: actuator usable stroke 2 (displ)
      | 11: actuator end cushion length 1 (displ)
      | 12: actuator end cushion length 2 (displ)
      | 13: actuator parasitic damping factor
      | 14: cross-chamber leakage factor (flow/press)
      | 15: ratio port openings according to area
      | 16: sample period (sec)
      |
      | Conversion factors used for converting
      | signals from external (user) to internal
      | (canonical) units:
      |
      | 17: displacement
      | 18: velocity
      | 19: force
      | 20: pressure
      | 21: flow
  note: Note: "1" and "2" denote actuator
      | cylinders on either side of the
      | actuator piston.  With positive
      | valve drive, oil is ported into
      | cylinder 1, resulting in positive
      | displacement.
  note: Auxiliary diagnostic output vector:
      | 1:   valve opening
      | 2:   C1 pressure
      | 3:   C2 pressure
      | 4:   delta pressure
      | 5:   force
      | 6:   velocity
      | 7:   C1 flow
      | 8:   C2 flow
      | 9:   total flow
      | 10: kinematic flow
      | 11: compressibility flow
      | 12: leakage flow
  cmd : Inport
  displ : Inport  Port=2
  veloc : Inport  Port=3
  spl press : Inport  Port=4
  rtn press : Inport  Port=5
  abs : Abs  SaturateOnIntegerOverflow=on
  actuator : S-Function  FunctionName=actuator  Parameters=actParamsA  SFunctionDeploymentMode=off  EnableBusSupport=off
  total flow sel : Selector  InputPortWidth=12  IndexOptions=Index vector (dialog)  Indices=9  OutputSizes=1
  force : Outport
  flow : Outport  Port=2
  wires:
  veloc/1 -> actuator/3
  displ/1 -> actuator/2
  actuator/1 -> force/1
  cmd/1 -> actuator/1
  rtn press/1 -> actuator/5
  spl press/1 -> actuator/4
  total flow sel/1 -> abs/1
  actuator/2 -> total flow sel/1
  abs/1 -> flow/1

== system OpenSeesPy_Simulink/MTS actuator/dynamic short channel #2/payload ==
  force : Inport
  Sum : Sum  Inputs=+----  InputSameDT=on  SaturateOnIntegerOverflow=on  OutDataTypeStr=Inherit: Same as first input
  damper : Gain  Gain=damperA*damperCanon  SaturateOnIntegerOverflow=on  OutDataTypeStr=Inherit: Same as input  ParamDataTypeStr=Inherit: Same as input
  div : Product  Inputs=*/  InputSameDT=on  SaturateOnIntegerOverflow=on  OutDataTypeStr=Inherit: Same as first input
  double integrator : Subsystem
  friction : Subsystem  mask{friction=frictionA*forceCanon, yieldDispl=yieldDisplA*lengthCanon, hysteresis=0}
      mask prompts: friction "Sliding friction"; yieldDispl "Equiv. yield displacement (in)"; hysteresis "Hysteresis constant"
  mass : Constant  Value=massA*massCanon
  static force : Constant  Value=staticForceA*forceCanon
  term1 : Terminator
  unit dly : UnitDelay  SampleTime=-1  HasFrameUpgradeWarning=on
  unit dly1 : UnitDelay  SampleTime=-1  HasFrameUpgradeWarning=on
  veloc units : Gain  Gain=1/velocCanon  SaturateOnIntegerOverflow=on  OutDataTypeStr=Inherit: Same as input  ParamDataTypeStr=Inherit: Same as input
  displ : Outport
  veloc : Outport  Port=2
  tag scope: ch2a=global
  wires:
  unit dly/1 -> [ch2a]
  [ch2b] -> Sum/3  "spring force"
  unit dly1/1 -> damper/1
  damper/1 -> Sum/4  "damper force"
  static force/1 -> Sum/5  "static force"
  double integrator/2(veloc) -> unit dly1/1, friction/1(veloc), veloc units/1
  double integrator/1(displ) -> unit dly/1, displ/1
  div/1 -> double integrator/1(accel)
  double integrator/3(acc) -> term1/1
  mass/1 -> div/2
  force/1 -> Sum/1  "total force"
  Sum/1 -> div/1  "inertial force"
  veloc units/1 -> veloc/1
  friction/1(force) -> Sum/2  "friction force"

== system OpenSeesPy_Simulink/MTS actuator/static channel #1/actuator//valve model ==
  note: Parameter vector:
      | 1:   oil bulk modulus (force/displ^2)
      | 2:   servovalve delay (sec)
      | 3:   servovalve overlap
      | 4:   rated pressure (force/displ^2)
      | 5:   rated flow at rated pressure (displ^3/sec)
      | 6:   nominal flow at rated pressure (displ^3/sec)
      | 7:   actuator piston area 1 (displ^2)
      | 8:   actuator piston area 2 (displ^2)
      | 9:   actuator usable stroke 1 (displ)
      | 10: actuator usable stroke 2 (displ)
      | 11: actuator end cushion length 1 (displ)
      | 12: actuator end cushion length 2 (displ)
      | 13: actuator parasitic damping factor
      | 14: cross-chamber leakage factor (flow/press)
      | 15: ratio port openings according to area
      | 16: sample period (sec)
      |
      | Conversion factors used for converting
      | signals from external (user) to internal
      | (canonical) units:
      |
      | 17: displacement
      | 18: velocity
      | 19: force
      | 20: pressure
      | 21: flow
  note: Auxiliary diagnostic output vector:
      | 1:   valve opening
      | 2:   C1 pressure
      | 3:   C2 pressure
      | 4:   delta pressure
      | 5:   force
      | 6:   velocity
      | 7:   C1 flow
      | 8:   C2 flow
      | 9:   total flow
      | 10: kinematic flow
      | 11: compressibility flow
      | 12: leakage flow
  note: Note: "1" and "2" denote actuator
      | cylinders on either side of the
      | actuator piston.  With positive
      | valve drive, oil is ported into
      | cylinder 1, resulting in positive
      | displacement.
  cmd : Inport
  displ : Inport  Port=2
  veloc : Inport  Port=3
  spl press : Inport  Port=4
  rtn press : Inport  Port=5
  abs : Abs  SaturateOnIntegerOverflow=on
  actuator : S-Function  FunctionName=actuator  Parameters=actParamsC  SFunctionDeploymentMode=off  EnableBusSupport=off
  total flow sel : Selector  InputPortWidth=12  IndexOptions=Index vector (dialog)  Indices=9  OutputSizes=1
  force : Outport
  flow : Outport  Port=2
  wires:
  abs/1 -> flow/1
  actuator/2 -> total flow sel/1
  total flow sel/1 -> abs/1
  spl press/1 -> actuator/4
  rtn press/1 -> actuator/5
  cmd/1 -> actuator/1
  actuator/1 -> force/1
  displ/1 -> actuator/2
  veloc/1 -> actuator/3

== system OpenSeesPy_Simulink/MTS actuator/static channel #1/payload ==
  force : Inport
  Sum : Sum  Inputs=+----  InputSameDT=on  SaturateOnIntegerOverflow=on  OutDataTypeStr=Inherit: Same as first input
  damper : Gain  Gain=damperC*damperCanon  SaturateOnIntegerOverflow=on  OutDataTypeStr=Inherit: Same as input  ParamDataTypeStr=Inherit: Same as input
  div : Product  Inputs=*/  InputSameDT=on  SaturateOnIntegerOverflow=on  OutDataTypeStr=Inherit: Same as first input
  double integrator : Subsystem
  friction : Subsystem  mask{friction=frictionC*forceCanon, yieldDispl=yieldDisplC*lengthCanon, hysteresis=0}
      mask prompts: friction "Sliding friction"; yieldDispl "Equiv. yield displacement (in)"; hysteresis "Hysteresis constant"
  mass : Constant  Value=massC*massCanon
  static force : Constant  Value=staticForceC*forceCanon
  term1 : Terminator
  unit dly : UnitDelay  SampleTime=-1  HasFrameUpgradeWarning=on
  unit dly1 : UnitDelay  SampleTime=-1  HasFrameUpgradeWarning=on
  veloc units : Gain  Gain=1/velocCanon  SaturateOnIntegerOverflow=on  OutDataTypeStr=Inherit: Same as input  ParamDataTypeStr=Inherit: Same as input
  displ : Outport
  veloc : Outport  Port=2
  tag scope: ch5a=global
  wires:
  unit dly/1 -> [ch5a]
  [ch5b] -> Sum/3  "spring force"
  unit dly1/1 -> damper/1
  damper/1 -> Sum/4  "damper force"
  static force/1 -> Sum/5  "static force"
  double integrator/2(veloc) -> unit dly1/1, friction/1(veloc), veloc units/1
  double integrator/1(displ) -> unit dly/1, displ/1
  div/1 -> double integrator/1(accel)
  double integrator/3(acc) -> term1/1
  mass/1 -> div/2
  force/1 -> Sum/1  "total force"
  Sum/1 -> div/1  "inertial force"
  veloc units/1 -> veloc/1
  friction/1(force) -> Sum/2  "friction force"

== system OpenSeesPy_Simulink/MTS actuator/static channel #2/actuator//valve model ==
  note: Parameter vector:
      | 1:   oil bulk modulus (force/displ^2)
      | 2:   servovalve delay (sec)
      | 3:   servovalve overlap
      | 4:   rated pressure (force/displ^2)
      | 5:   rated flow at rated pressure (displ^3/sec)
      | 6:   nominal flow at rated pressure (displ^3/sec)
      | 7:   actuator piston area 1 (displ^2)
      | 8:   actuator piston area 2 (displ^2)
      | 9:   actuator usable stroke 1 (displ)
      | 10: actuator usable stroke 2 (displ)
      | 11: actuator end cushion length 1 (displ)
      | 12: actuator end cushion length 2 (displ)
      | 13: actuator parasitic damping factor
      | 14: cross-chamber leakage factor (flow/press)
      | 15: ratio port openings according to area
      | 16: sample period (sec)
      |
      | Conversion factors used for converting
      | signals from external (user) to internal
      | (canonical) units:
      |
      | 17: displacement
      | 18: velocity
      | 19: force
      | 20: pressure
      | 21: flow
  note: Note: "1" and "2" denote actuator
      | cylinders on either side of the
      | actuator piston.  With positive
      | valve drive, oil is ported into
      | cylinder 1, resulting in positive
      | displacement.
  note: Auxiliary diagnostic output vector:
      | 1:   valve opening
      | 2:   C1 pressure
      | 3:   C2 pressure
      | 4:   delta pressure
      | 5:   force
      | 6:   velocity
      | 7:   C1 flow
      | 8:   C2 flow
      | 9:   total flow
      | 10: kinematic flow
      | 11: compressibility flow
      | 12: leakage flow
  cmd : Inport
  displ : Inport  Port=2
  veloc : Inport  Port=3
  spl press : Inport  Port=4
  rtn press : Inport  Port=5
  abs : Abs  SaturateOnIntegerOverflow=on
  actuator : S-Function  FunctionName=actuator  Parameters=actParamsC  SFunctionDeploymentMode=off  EnableBusSupport=off
  total flow sel : Selector  InputPortWidth=12  IndexOptions=Index vector (dialog)  Indices=9  OutputSizes=1
  force : Outport
  flow : Outport  Port=2
  wires:
  veloc/1 -> actuator/3
  displ/1 -> actuator/2
  actuator/1 -> force/1
  cmd/1 -> actuator/1
  rtn press/1 -> actuator/5
  spl press/1 -> actuator/4
  total flow sel/1 -> abs/1
  actuator/2 -> total flow sel/1
  abs/1 -> flow/1

== system OpenSeesPy_Simulink/MTS actuator/static channel #2/payload ==
  force : Inport
  Sum : Sum  Inputs=+----  InputSameDT=on  SaturateOnIntegerOverflow=on  OutDataTypeStr=Inherit: Same as first input
  damper : Gain  Gain=damperC*damperCanon  SaturateOnIntegerOverflow=on  OutDataTypeStr=Inherit: Same as input  ParamDataTypeStr=Inherit: Same as input
  div : Product  Inputs=*/  InputSameDT=on  SaturateOnIntegerOverflow=on  OutDataTypeStr=Inherit: Same as first input
  double integrator : Subsystem
  friction : Subsystem  mask{friction=frictionC*forceCanon, yieldDispl=yieldDisplC*lengthCanon, hysteresis=0}
      mask prompts: friction "Sliding friction"; yieldDispl "Equiv. yield displacement (in)"; hysteresis "Hysteresis constant"
  mass : Constant  Value=massC*massCanon
  static force : Constant  Value=staticForceC*forceCanon
  term1 : Terminator
  unit dly : UnitDelay  SampleTime=-1  HasFrameUpgradeWarning=on
  unit dly1 : UnitDelay  SampleTime=-1  HasFrameUpgradeWarning=on
  veloc units : Gain  Gain=1/velocCanon  SaturateOnIntegerOverflow=on  OutDataTypeStr=Inherit: Same as input  ParamDataTypeStr=Inherit: Same as input
  displ : Outport
  veloc : Outport  Port=2
  tag scope: ch6a=global
  wires:
  unit dly/1 -> [ch6a]
  [ch6b] -> Sum/3  "spring force"
  unit dly1/1 -> damper/1
  damper/1 -> Sum/4  "damper force"
  static force/1 -> Sum/5  "static force"
  double integrator/2(veloc) -> unit dly1/1, friction/1(veloc), veloc units/1
  double integrator/1(displ) -> unit dly/1, displ/1
  div/1 -> double integrator/1(accel)
  double integrator/3(acc) -> term1/1
  mass/1 -> div/2
  force/1 -> Sum/1  "total force"
  Sum/1 -> div/1  "inertial force"
  veloc units/1 -> veloc/1
  friction/1(force) -> Sum/2  "friction force"

== system OpenSeesPy_Simulink/MTS actuator/static channel #3/actuator//valve model ==
  note: Parameter vector:
      | 1:   oil bulk modulus (force/displ^2)
      | 2:   servovalve delay (sec)
      | 3:   servovalve overlap
      | 4:   rated pressure (force/displ^2)
      | 5:   rated flow at rated pressure (displ^3/sec)
      | 6:   nominal flow at rated pressure (displ^3/sec)
      | 7:   actuator piston area 1 (displ^2)
      | 8:   actuator piston area 2 (displ^2)
      | 9:   actuator usable stroke 1 (displ)
      | 10: actuator usable stroke 2 (displ)
      | 11: actuator end cushion length 1 (displ)
      | 12: actuator end cushion length 2 (displ)
      | 13: actuator parasitic damping factor
      | 14: cross-chamber leakage factor (flow/press)
      | 15: ratio port openings according to area
      | 16: sample period (sec)
      |
      | Conversion factors used for converting
      | signals from external (user) to internal
      | (canonical) units:
      |
      | 17: displacement
      | 18: velocity
      | 19: force
      | 20: pressure
      | 21: flow
  note: Auxiliary diagnostic output vector:
      | 1:   valve opening
      | 2:   C1 pressure
      | 3:   C2 pressure
      | 4:   delta pressure
      | 5:   force
      | 6:   velocity
      | 7:   C1 flow
      | 8:   C2 flow
      | 9:   total flow
      | 10: kinematic flow
      | 11: compressibility flow
      | 12: leakage flow
  note: Note: "1" and "2" denote actuator
      | cylinders on either side of the
      | actuator piston.  With positive
      | valve drive, oil is ported into
      | cylinder 1, resulting in positive
      | displacement.
  cmd : Inport
  displ : Inport  Port=2
  veloc : Inport  Port=3
  spl press : Inport  Port=4
  rtn press : Inport  Port=5
  abs : Abs  SaturateOnIntegerOverflow=on
  actuator : S-Function  FunctionName=actuator  Parameters=actParamsC  SFunctionDeploymentMode=off  EnableBusSupport=off
  total flow sel : Selector  InputPortWidth=12  IndexOptions=Index vector (dialog)  Indices=9  OutputSizes=1
  force : Outport
  flow : Outport  Port=2
  wires:
  abs/1 -> flow/1
  actuator/2 -> total flow sel/1
  total flow sel/1 -> abs/1
  spl press/1 -> actuator/4
  rtn press/1 -> actuator/5
  cmd/1 -> actuator/1
  actuator/1 -> force/1
  displ/1 -> actuator/2
  veloc/1 -> actuator/3
